simulink model "Smart_City_QCar2_VIRTUAL_car4"  (R2024b)
settings: Solver=ode1  StartTime=0.0  StopTime=inf  FixedStep=Controller_Sample_Time  RelTol=1e-3  EnableMultiTasking=on
values from neighbouring files (symbols this model uses):
  Audio_Sample_Time = 0.3    [Setup_QCar1and2_params.m]
  cameraStepSize = 3e-2    (= 0.03)    [Setup_QCar1and2_params.m]
  CSI_Sample_Time = 1/60    (= 0.0166666666667)    [Setup_QCar1and2_params.m]
  ImageDisplay_Sample_Time = CSI_Sample_Time*6    (= 0.1)    [Setup_QCar1and2_params.m]
  Initialization_Time = 5    [Setup_QCar1and2_params.m]
  LiDAR_Sample_Time = CSI_Sample_Time*3    (= 0.05)    [Setup_QCar1and2_params.m]
  map_mask = [1 1 1 0 0 1 0]    [Setup_QCar1and2_params.m]
  NN_Sample_Time = RealSense_Sample_Time*1    (= 0.0333333333333)    [Setup_QCar1and2_params.m]
  path_x = [0.826 0.836 0.846 0.856 0.866 0.876 0.886 0.896 0.906 0.916 0.926 0.936 ... (740 elements, 740x1)]    [SDCS_Paths_7.mat]
  path_x2 = [-0.614 -0.604 -0.594 -0.584 -0.574 -0.564 -0.554 -0.544 -0.534 -0.524 -0.514 -0.504 ... (1090 elements, 1090x1)]    [SDCS_Paths_7.mat]
  path_x3 = [-0.614 -0.603821428571 -0.593642857143 -0.583464285714 -0.573285714286 -0.563107142857 -0.552928571429 -0.54275 -0.532571428571 -0.522392857143 -0.512214285714 -0.502035714286 ... (714 elements, 714x1)]    [SDCS_Paths_7.mat]
  path_x4 = [-0.614 -0.604 -0.594 -0.584 -0.574 -0.564 -0.554 -0.544 -0.534 -0.524 -0.514 -0.504 ... (1761 elements, 1761x1)]    [SDCS_Paths_7.mat]
  path_x5 = [1.436 1.42588571429 1.41577142857 1.40565714286 1.39554285714 1.38542857143 1.37531428571 1.3652 1.35508571429 1.34497142857 1.33485714286 1.32474285714 ... (574 elements, 574x1)]    [SDCS_Paths_7.mat]
  path_x6 = [1.436 1.42588571429 1.41577142857 1.40565714286 1.39554285714 1.38542857143 1.37531428571 1.3652 1.35508571429 1.34497142857 1.33485714286 1.32474285714 ... (1288 elements, 1288x1)]    [SDCS_Paths_7.mat]
  path_x7 = [-1.5778487585 -1.56959877056 -1.56127865467 -1.55288878259 -1.54442952915 -1.53590127231 -1.52730439309 -1.51863927561 -1.50990630701 -1.50110587746 -1.49223838016 -1.4833042113 ... (2260 elements, 2260x1)]    [SDCS_Paths_7.mat]
  path_y = [-1.0887 -1.0887 -1.0887 -1.0887 -1.0887 -1.0887 -1.0887 -1.0887 -1.0887 -1.0887 -1.0887 -1.0887 ... (740 elements, 740x1)]    [SDCS_Paths_7.mat]
  path_y2 = [-1.0887 -1.0887 -1.0887 -1.0887 -1.0887 -1.0887 -1.0887 -1.0887 -1.0887 -1.0887 -1.0887 -1.0887 ... (1090 elements, 1090x1)]    [SDCS_Paths_7.mat]
  path_y3 = [-1.0887 -1.0887 -1.0887 -1.0887 -1.0887 -1.0887 -1.0887 -1.0887 -1.0887 -1.0887 -1.0887 -1.0887 ... (714 elements, 714x1)]    [SDCS_Paths_7.mat]
  path_y4 = [-1.0887 -1.0887 -1.0887 -1.0887 -1.0887 -1.0887 -1.0887 -1.0887 -1.0887 -1.0887 -1.0887 -1.0887 ... (1761 elements, 1761x1)]    [SDCS_Paths_7.mat]
  path_y5 = [-0.8157 -0.8157 -0.8157 -0.8157 -0.8157 -0.8157 -0.8157 -0.8157 -0.8157 -0.8157 -0.8157 -0.8157 ... (574 elements, 574x1)]    [SDCS_Paths_7.mat]
  path_y6 = [-0.8157 -0.8157 -0.8157 -0.8157 -0.8157 -0.8157 -0.8157 -0.8157 -0.8157 -0.8157 -0.8157 -0.8157 ... (1288 elements, 1288x1)]    [SDCS_Paths_7.mat]
  path_y7 = [-0.614490295955 -0.61974988896 -0.624981792226 -0.630185771997 -0.635361595765 -0.640509032279 -0.645627851559 -0.6507178249 -0.655778724888 -0.660810325409 -0.665812401655 -0.670784730139 ... (2260 elements, 2260x1)]    [SDCS_Paths_7.mat]
  RealSense_Sample_Time = CSI_Sample_Time*2    (= 0.0333333333333)    [Setup_QCar1and2_params.m]
undefined symbols (not defined in the file or in its folder): DiscIntNeverNeededParam, gcbh, Joystick_Sample_Time, JPEG, qc_get_step_size, video_display_show
libraries: quarc_library x61, simulink_extras x9, simulink x5
(part 1 of 4)
settings Model: SimulationMode=external  ExtModeTrigDuration=10000  Creator=PKaram  LastModifiedBy=user
settings SolverCC: AlgebraicLoopSolver=TrustRegion  PositivePriorityOrder=on  AutoInsertRateTranBlk=on
settings DataIOCC: ReturnWorkspaceOutputs=off
settings DebuggingCC: ParameterPrecisionLossMsg=none  UnconnectedInputMsg=warning  UnconnectedOutputMsg=warning  UnconnectedLineMsg=warning  ArithmeticOperatorsInVariantConditions=warning
settings ModelReferenceCC: EnableRefExpFcnMdlSchedulingChecks=on
settings SFSimCC: SimUseLocalCustomCode=off  CustomCodeUndefinedFunction=UseInterfaceOnly
settings RTWCC: Description=QUARC Win64 Target Using Toolchain  SystemTargetFile=quarc_win64.tlc  TemplateMakefile=quarc_linux_nvidia_tmf  RTWUseLocalCustomCode=off  Toolchain=QUARC win64 | nmake (64-bit Windows)  BuildConfiguration=Faster Runs  GPUComputeCapability=3.5  DLArmComputeVersion=19.05
settings CodeAppCC: StateflowObjectComments=on
settings STFCustomTargetCC: TargetLangStandard=C99 (ISO)  ConcurrentExecutionCompliant=on  GRTInterface=on  UseToolchainInfoCompliant=on  SystemTargetFile=quarc_win64.tlc
settings GRTTargetCC: ParMdlRefBuildCompliant=off  CompOptLevelCompliant=off  CombineOutputUpdateFcns=off  MatFileLogging=off  CPPClassGenCompliant=off  GRTInterface=on  ExtMode=on  ExtModeMexFile=quarc_comm  ExtModeMexArgs='-w -d %d -uri %u -car_number 4','shmem://%m:1'
settings ConfigComp: CovMetricSettings=dswe

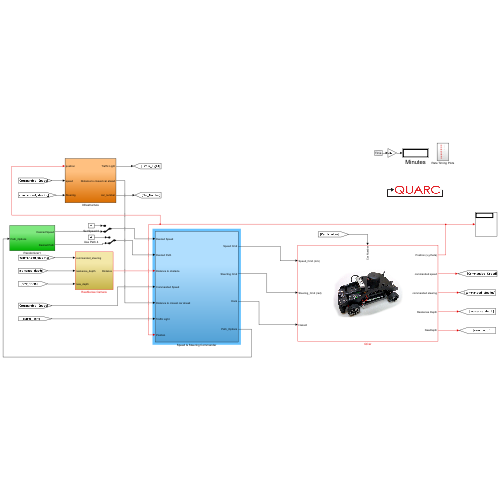
[thumbnail: Simulink's stored preview of the top-level diagram]
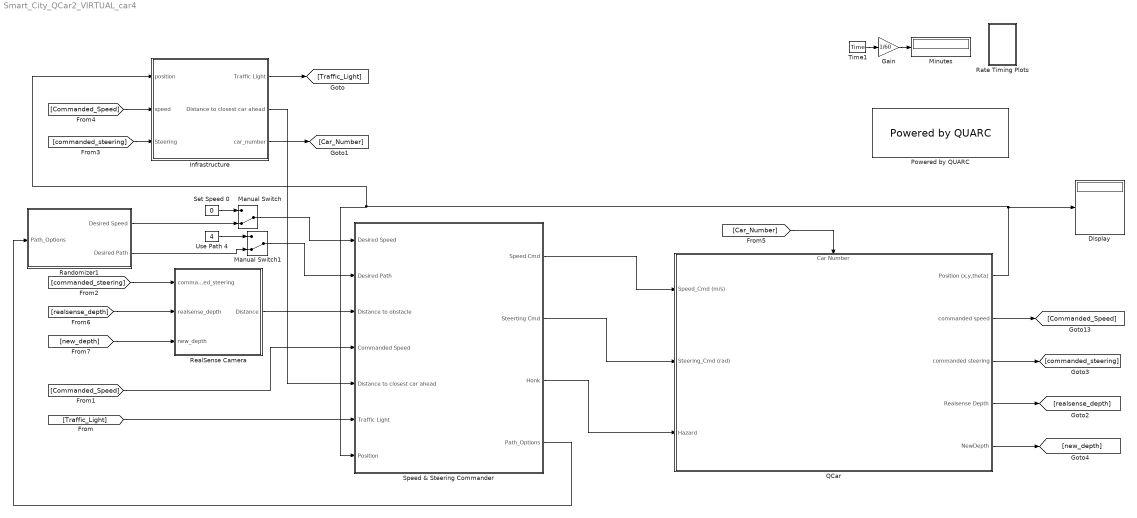
== system Smart_City_QCar2_VIRTUAL_car4 ==
  Display : Display
  Gain : Gain  Gain=1/60
  Infrastructure : Subsystem
  Manual Switch : ManualSwitch  CurrentSetting=0
  Manual Switch1 : ManualSwitch  CurrentSetting=0
  Minutes : Display
  Powered by QUARC : quarc_library/Logos/Powered by QUARC
  QCar : Subsystem
      settings: PortSchema="{\"entries\":[{\"content\":{\"sides\":[{\"content\":{\"connectorIds\":[\"In1\",\"In2\",\"In3\"]},\"type\":\"ConnectorPlacement.EquallySpacedRectSide\",\"uuid\":\"02a1560c-0405-4b97-a286-7d926425b90e\"},{\"content\":{\"connectorIds\":[\"Out1\",\"Out2\",\"Out3\",\"Out4\",\"Out5\"],\"side\":\"RIGHT\"},\"type\":\"ConnectorPlacement.EquallySpacedRectSide\",\"uuid\":\"39c5c8b2-4245-4ec7-b5b3-4c98e6a2673a\"},{\"content\":{\"connectorIds\":[\"In4\"],\"side\":\"TOP\"},\"type\":\"ConnectorPlacement.EquallySpacedRectSide\",\"uuid\":\"1752f2f8-f0ed-4d28-b225-c74112047425\"}]},\"type\":\"ConnectorPlacement.EquallySpacedConnector\",\"uuid\":\"d58cf7e2-2005-4c93-8747-d53ee0601380\"}],\"packageUris\":[\"http://schema.mathworks.com/mf0/Connector/R2020b\"],\"version\":\"1.0\"}"
      mask Display: image('QCar.png', [0,0,0,0,50,50]);
  Randomizer1 : Subsystem
  Rate Timing Plots : Subsystem
  RealSense Camera : Subsystem
  Set Speed 0 : Constant  Value=0
  Speed & Steering Commander : Subsystem
  Time1 : quarc_library/Sources/Time/Time  time_source=Wall clock  sample_time=qc_get_step_size
  Use Path 4 : Constant  Value=4
  wires:
  [commanded_steering] -> RealSense Camera/1(commanded_steering)
  [commanded_steering] -> Infrastructure/3(Steering)
  Use Path 4/1 -> Manual Switch1/1
  QCar/1(Position (x,y,theta)) -> Speed & Steering Commander/7(Position), Infrastructure/1(position), Display/1
  [Traffic_Light] -> Speed & Steering Commander/6(Traffic Light)
  QCar/3(commanded steering) -> [commanded_steering]
  Randomizer1/1(Desired Speed) -> Manual Switch/2
  [Commanded_Speed] -> Speed & Steering Commander/4(Commanded Speed)
  Time1/1 -> Gain/1
  Manual Switch/1 -> Speed & Steering Commander/1(Desired Speed)
  Manual Switch1/1 -> Speed & Steering Commander/2(Desired Path)
  Speed & Steering Commander/2(Steerting Cmd) -> QCar/2(Steering_Cmd (rad))
  Infrastructure/2(Distance to closest car ahead) -> Speed & Steering Commander/5(Distance to closest car ahead)
  Speed & Steering Commander/1(Speed Cmd) -> QCar/1(Speed_Cmd (m/s))
  Speed & Steering Commander/4(Path_Options) -> Randomizer1/1(Path_Options)
  Speed & Steering Commander/3(Honk) -> QCar/3(Hazard)
  Infrastructure/3(car_number) -> [Car_Number]
  QCar/2(commanded speed) -> [Commanded_Speed]
  Set Speed 0/1 -> Manual Switch/1
  [Commanded_Speed] -> Infrastructure/2("speed ")
  Randomizer1/2(Desired Path) -> Manual Switch1/2
  Gain/1 -> Minutes/1
  RealSense Camera/1(Distance) -> Speed & Steering Commander/3(Distance to obstacle)
  [Car_Number] -> QCar/4(Car Number)
  QCar/4(Realsense Depth) -> [realsense_depth]
  [realsense_depth] -> RealSense Camera/2(realsense_depth)
  QCar/5(NewDepth) -> [new_depth]
  [new_depth] -> RealSense Camera/3(new_depth)
  Infrastructure/1(Traffic Light) -> [Traffic_Light]

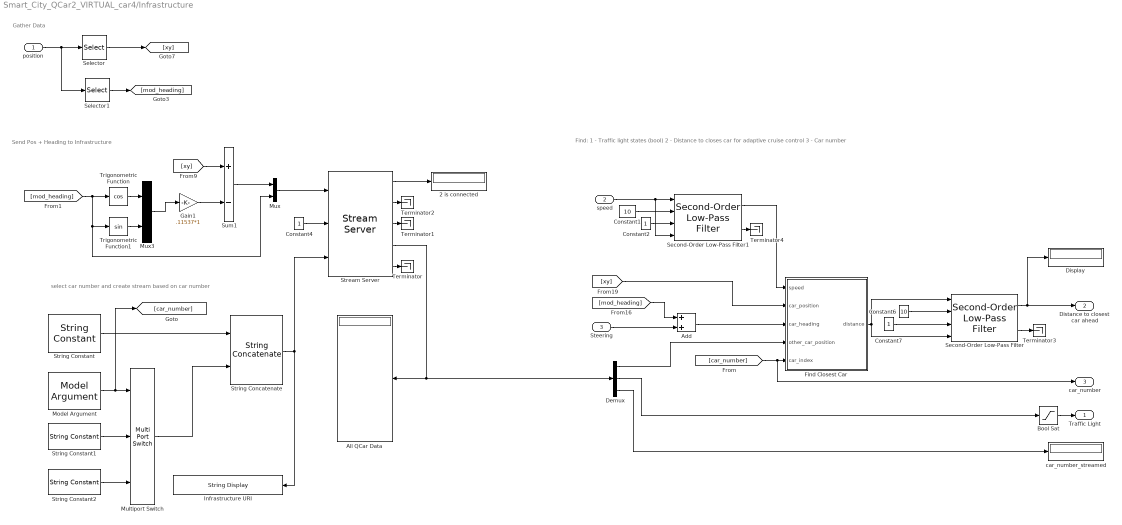
== system Smart_City_QCar2_VIRTUAL_car4/Infrastructure ==
  note: select car number and create stream based on car number
  note: Find:
      | 1 - Traffic light states (bool)
      | 2 - Distance to closes car for adaptive cruise control
      | 3 - Car number
  note: Send Pos + Heading to Infrastructure
  note: Gather Data
  position : Inport
  "speed " : Inport  Port=2
  Steering : Inport  Port=3
  2 is connected : Display
      settings: Decimation=100
  Add : Sum
  All QCar Data : Display
  Bool Sat : Saturate  UpperLimit=1  LowerLimit=0
  Constant1 : Constant  Value=10
  Constant2 : Constant
  Constant4 : Constant
  Constant6 : Constant  Value=10
  Constant7 : Constant
  Demux : Demux  Outputs=[10 1 1]
  Display : Display
  Find Closest Car : Subsystem
  Gain1 : Gain  Gain=.11537*1
  Infrastructure URI : quarc_library/Strings/String Display  alignment=center  display_mode=Single line  sample_time=-1  use_new=off
      settings: SourceProductName=QUARC Targets
  Model Argument : quarc_library/Sources/Signals/Model Argument  argument_name=car_number  has_value=on  data_type_mode=Specify via dialog  data_type=uint8  max_length=80  default_value=0  default_string=4  variable_size=on
      settings: AttributesFormatString=(-%<argument_name>)  SourceProductName=QUARC Targets
  Multiport Switch : MultiPortSwitch  DataPortOrder=Specify indices  DataPortIndices={4,5}  SaturateOnIntegerOverflow=off  InputSameDT=off
  Mux : Mux  Inputs=2
  Mux3 : Mux  Inputs=2
  Second-Order Low-Pass Filter : quarc_library/Continuous/Second-Order Low-Pass Filter  params_source=External (input ports)  input_width=1  input_zeta=1  input_init=0
  Second-Order Low-Pass Filter1 : quarc_library/Continuous/Second-Order Low-Pass Filter  params_source=External (input ports)  input_width=1  input_zeta=1  input_init=0
  Selector : Selector  InputPortWidth=3  IndexOptions=Index vector (dialog)  Indices=1:2  OutputSizes=1
  Selector1 : Selector  InputPortWidth=3  IndexOptions=Index vector (dialog)  Indices=3  OutputSizes=1
  Stream Server : quarc_library/Communications/Basic/Stream Server  uri_source=External input port  uri=tcpip://localhost:4444?nagle='off'  send_buffer_size=1460  receive_buffer_size=1460  byte_order=little endian (Intel - LSB first)  optimization=Minimum latency  send_options=Send most recent data  receive_options=Receive most recent data  default_value=10* ones (1,12)  sample_time=qc_get_step_size  active=off  implementation=Use blocking I/O in a separate thread  send_fifo_size=1  receive_fifo_size=1  send_priority=0  receive_priority=0  send_dimensions=off  receive_dimensions=off  max_dimensions=-1  data_type=Inherited via back propagation  type_expr=BusObject
  String Concatenate : quarc_library/Strings/String Concatenate  num_inputs=2  max_length=0  output_size=Inherit from input
      settings: SourceProductName=QUARC Targets
  String Constant : quarc_library/Strings/String Constant  string_value=tcpip://localhost:  evaluate_string=off  string_type=text  max_length=80  sample_time=inf  variable_size=off
      settings: AttributesFormatString="\"tcpip://localhost:\""  SourceProductName=QUARC Targets
  String Constant1 : quarc_library/Strings/String Constant  string_value=4444  evaluate_string=off  string_type=text  max_length=80  sample_time=inf  variable_size=off
      settings: AttributesFormatString="\"4444\""  SourceProductName=QUARC Targets
  String Constant2 : quarc_library/Strings/String Constant  string_value=5555  evaluate_string=off  string_type=text  max_length=80  sample_time=inf  variable_size=off
      settings: AttributesFormatString="\"5555\""  SourceProductName=QUARC Targets
  Sum1 : Sum  Inputs=+-
  Terminator{,1..4} (5 alike) : Terminator
  Trigonometric Function : Trigonometry  Operator=cos
  Trigonometric Function1 : Trigonometry
  car_number_streamed : Display
  Traffic Light : Outport
  Distance to closest car ahead : Outport  Port=2
  car_number : Outport  Port=3
  wires:
  Constant7/1 -> Second-Order Low-Pass Filter/3
  Constant4/1 -> Stream Server/2
  Stream Server/1 -> 2 is connected/1
  Constant6/1 -> Second-Order Low-Pass Filter/2
  position/1 -> Selector1/1, Selector/1
  Selector/1 -> [xy]
  Selector1/1 -> [mod_heading]
  Second-Order Low-Pass Filter/1 -> Display/1, Distance to closest car ahead/1
  Constant1/1 -> Second-Order Low-Pass Filter1/2
  "speed "/1 -> Second-Order Low-Pass Filter1/4, Second-Order Low-Pass Filter1/1
  Stream Server/4 -> All QCar Data/1, Demux/1
  [xy] -> Find Closest Car/2(car_position)
  Constant2/1 -> Second-Order Low-Pass Filter1/3
  Second-Order Low-Pass Filter1/1 -> Find Closest Car/1("speed ")
  Find Closest Car/1(distance) -> Second-Order Low-Pass Filter/1, Second-Order Low-Pass Filter/4
  Add/1 -> Find Closest Car/3(car_heading)
  [mod_heading] -> Add/1
  Steering/1 -> Add/2
  Demux/1 -> Find Closest Car/4(other_car_position)
  Demux/2 -> Bool Sat/1
  Bool Sat/1 -> Traffic Light/1
  Mux/1 -> Stream Server/1
  Sum1/1 -> Mux/1
  Demux/3 -> car_number_streamed/1
  [mod_heading] -> Mux/2, Trigonometric Function1/1, Trigonometric Function/1
  Mux3/1 -> Gain1/1
  Trigonometric Function1/1 -> Mux3/2
  [xy] -> Sum1/1
  Gain1/1 -> Sum1/2
  Trigonometric Function/1 -> Mux3/1
  Stream Server/5 -> Terminator/1
  Stream Server/3 -> Terminator1/1
  Stream Server/2 -> Terminator2/1
  Second-Order Low-Pass Filter/2 -> Terminator3/1
  Second-Order Low-Pass Filter1/2 -> Terminator4/1
  String Constant/1 -> String Concatenate/1
  Model Argument/1 -> [car_number], Multiport Switch/1
  String Constant1/1 -> Multiport Switch/2
  String Constant2/1 -> Multiport Switch/3
  Multiport Switch/1 -> String Concatenate/2
  String Concatenate/1 -> Stream Server/3, Infrastructure URI/1
  [car_number] -> car_number/1, Find Closest Car/5(car_index)

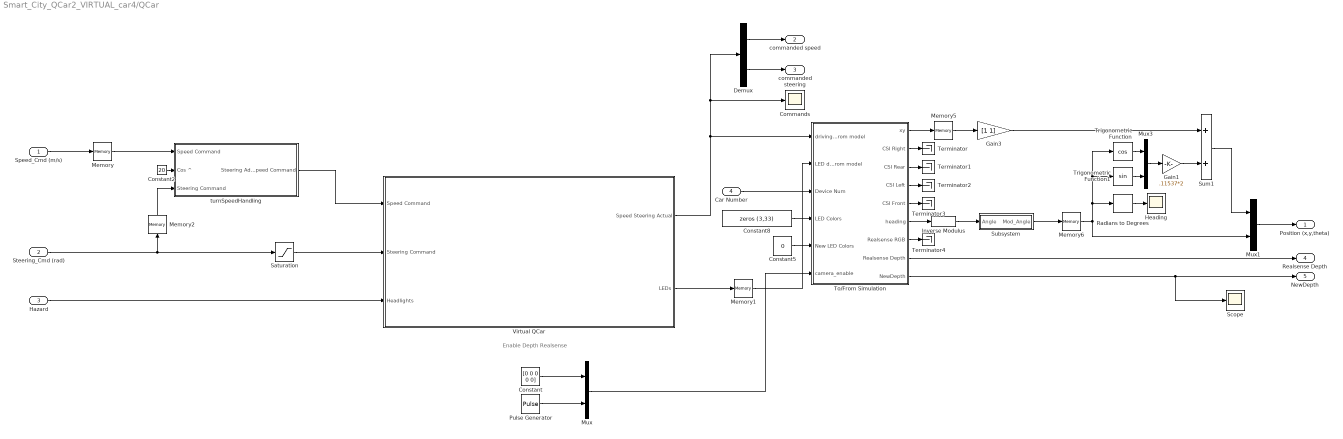
== system Smart_City_QCar2_VIRTUAL_car4/QCar ==
  note: Enable Depth Realsense
  Speed_Cmd (m/s) : Inport
  Steering_Cmd (rad) : Inport  Port=2
  Hazard : Inport  Port=3
  Car Number : Inport  Port=4
  Commands : Scope
  Constant : Constant  Value=[0 0 0 0 0]  SampleTime=RealSense_Sample_Time
  Constant2 : Constant  Value=20
  Constant5 : Constant  Value=0
  Constant8 : Constant  Value=zeros (3,33)
  Demux : Demux  Outputs=2
  Gain1 : Gain  Gain=.11537*2
  Gain3 : Gain  Gain=[1 1]
  Heading : Scope
  Inverse Modulus : quarc_library/Discontinuities/Inverse Modulus  modulus=2*pi  output_derivative=off  output_revolutions=off  max_x=Inf  min_x=-Inf
  Memory : Memory
  Memory1 : Memory  InitialCondition=zeros (1,16)  InheritSampleTime=on  LinearizeMemory=on  LinearizeAsDelay=on
  Memory2 : Memory  InheritSampleTime=on  LinearizeMemory=on  LinearizeAsDelay=on
  Memory5 : Memory  InitialCondition=[0 0]  InheritSampleTime=on  LinearizeMemory=on  LinearizeAsDelay=on
  Memory6 : Memory  InheritSampleTime=on  LinearizeMemory=on  LinearizeAsDelay=on
  Mux : Mux  Inputs=2
  Mux1 : Mux  Inputs=2
  Mux3 : Mux  Inputs=2
  Pulse Generator : DiscretePulseGenerator  SampleTime=RealSense_Sample_Time
  Radians to Degrees : simulink_extras/Transformations/Radians to Degrees
  Saturation : Saturate  UpperLimit=0.6  LowerLimit=-0.6
  Scope : Scope
  Subsystem : Subsystem
  Sum1 : Sum
  Terminator{,1..4} (5 alike) : Terminator
  To/From Simulation : Subsystem
  Trigonometric Function : Trigonometry  Operator=cos
  Trigonometric Function1 : Trigonometry
  Virtual QCar : Subsystem
  turnSpeedHandling : Subsystem
  Position (x,y,theta) : Outport
  commanded speed : Outport  Port=2
  commanded steering : Outport  Port=3
  Realsense Depth : Outport  Port=4
  NewDepth : Outport  Port=5
  wires:
  Saturation/1 -> Virtual QCar/2(Steering Command)
  Memory6/1 -> Mux1/2, Trigonometric Function/1, Trigonometric Function1/1, Radians to Degrees/1
  Subsystem/1(Mod_Angle) -> Memory6/1
  Memory5/1 -> Gain3/1
  turnSpeedHandling/1(Steering Adjusted Speed Command) -> Virtual QCar/1(Speed Command)
  Hazard/1 -> Virtual QCar/3(Headlights)
  Mux1/1 -> Position (x,y,theta)/1
  Sum1/1 -> Mux1/1
  Memory2/1 -> turnSpeedHandling/3(Steering Command)
  Constant2/1 -> turnSpeedHandling/2(Cos ^)
  Car Number/1 -> To/From Simulation/3(Device Num)
  Gain3/1 -> Sum1/1
  Gain1/1 -> Sum1/2
  Mux3/1 -> Gain1/1
  Trigonometric Function1/1 -> Mux3/2
  Trigonometric Function/1 -> Mux3/1
  Radians to Degrees/1 -> Heading/1
  Inverse Modulus/1 -> Subsystem/1(Angle)
  Virtual QCar/1(Speed Steering Actual) -> Demux/1, Commands/1, To/From Simulation/1(driving data from model)
  Virtual QCar/2(LEDs) -> Memory1/1
  Demux/1 -> commanded speed/1
  Constant8/1 -> To/From Simulation/4(LED Colors)
  Constant5/1 -> To/From Simulation/5(New LED Colors)
  To/From Simulation/6(heading) -> Inverse Modulus/1
  To/From Simulation/1(xy) -> Memory5/1
  Memory1/1 -> To/From Simulation/2(LED data from model)
  To/From Simulation/8(Realsense Depth) -> Realsense Depth/1
  Speed_Cmd (m/s)/1 -> Memory/1
  Memory/1 -> turnSpeedHandling/1(Speed Command)
  Steering_Cmd (rad)/1 -> Memory2/1, Saturation/1
  To/From Simulation/2(CSI Right) -> Terminator/1
  To/From Simulation/3(CSI Rear) -> Terminator1/1
  To/From Simulation/4(CSI Left) -> Terminator2/1
  To/From Simulation/5(CSI Front) -> Terminator3/1
  To/From Simulation/7(Realsense RGB) -> Terminator4/1
  Demux/2 -> commanded steering/1
  Constant/1 -> Mux/1
  Mux/1 -> To/From Simulation/6(camera_enable)
  To/From Simulation/9(NewDepth) -> Scope/1, NewDepth/1
  Pulse Generator/1 -> Mux/2

== system Smart_City_QCar2_VIRTUAL_car4/Randomizer1 ==
  note: Tunable Params
  Path_Options : Inport
  Base Speed : Constant  Value=.35
  Display : Display
  Display1 : Display
  MATLAB Function : MATLAB Function  TreatAsAtomicUnit=on
  Manual Map Mask : Gain  Gain=[1 1 1 1 1 1 0]
  Memory1 : Memory  InitialCondition=2  InheritSampleTime=on  LinearizeMemory=on  LinearizeAsDelay=on
  Memory2 : Memory  InitialCondition=1  InheritSampleTime=on  LinearizeMemory=on  LinearizeAsDelay=on
  Path 4 : Constant  Value=4
  Start on path 4 : Switch  Criteria=u2 > Threshold  Threshold=8  SaturateOnIntegerOverflow=off  InputSameDT=off
  Subsystem1 : Subsystem
  Terminator : Terminator
  Time : quarc_library/Sources/Time/Time  time_source=Wall clock  sample_time=qc_get_step_size
  Time b/w Path Changes : Constant  Value=3
  Desired Speed : Outport
  Desired Path : Outport  Port=2
  wires:
  Memory1/1 -> MATLAB Function/1(Previous_Path)
  Memory2/1 -> MATLAB Function/2(Previous_Speed)
  Time b/w Path Changes/1 -> Subsystem1/1(Random Period)
  Subsystem1/1(RisingEdgeTrigger) -> MATLAB Function/5(randomize)
  Base Speed/1 -> MATLAB Function/4(Speed_Cmd_Base)
  MATLAB Function/2(Desired_Speed) -> Desired Speed/1, Memory2/1, Display1/1
  MATLAB Function/1(Desired_Path) -> Start on path 4/1, Memory1/1
  Path_Options/1 -> Manual Map Mask/1
  MATLAB Function/3(Accel_Limit) -> Terminator/1
  Time/1 -> Start on path 4/2
  Start on path 4/1 -> Display/1, Desired Path/1
  Path 4/1 -> Start on path 4/3
  Manual Map Mask/1 -> MATLAB Function/3(Path_Options)

== system Smart_City_QCar2_VIRTUAL_car4/Rate Timing Plots ==
  Audio : Scope
  CSI : Scope
  Control : Scope
  Image Displays : Scope
  Joystick : Scope  Commented=on
  LCD : Scope
  LiDAR : Scope
  NN Rate : Scope
  RealSense : Scope
  monitorTiming : Subsystem
  monitorTiming1 : Subsystem
  monitorTiming2 : Subsystem
  monitorTiming3 : Subsystem
  monitorTiming4 : Subsystem  Commented=on
  monitorTiming5 : Subsystem
  monitorTiming6 : Subsystem
  monitorTiming7 : Subsystem
  monitorTiming8 : Subsystem
  wires:
  monitorTiming/1(Timing (s)) -> CSI/1
  monitorTiming1/1(Timing (s)) -> Control/1
  monitorTiming3/1(Timing (s)) -> Image Displays/1
  monitorTiming4/1(Timing (s)) -> Joystick/1
  monitorTiming2/1(Timing (s)) -> RealSense/1
  monitorTiming5/1(Timing (s)) -> LiDAR/1
  monitorTiming6/1(Timing (s)) -> NN Rate/1
  monitorTiming7/1(Timing (s)) -> LCD/1
  monitorTiming8/1(Timing (s)) -> Audio/1

== system Smart_City_QCar2_VIRTUAL_car4/RealSense Camera ==
  note: Capture Realsense and do Object Detection
  commanded_steering : Inport
  realsense_depth : Inport  Port=2
  new_depth : Inport  Port=3
  Constant8 : Constant  Value=50
  Constant9 : Constant
  Distance to Object Detected : Display
  Gain : Gain  Gain=3.9/255
  Image Transform : quarc_library/Image Processing/Generic/Image Transform  algorithm=Colorize  color_theme=KRYGCBMW  min_pixel=0  max_pixel=5  contour_depth=1  focal_length=308  principal_point=[262 334]  radial_coeffs=[-0.3129 0.0907]  tangential_coeffs=[]  extrapolated_pixel=0  interpolation=nearest  row_coords=0  column_coords=0  output_height=480  output_width=640  angle=0  origin=[240 320]  output_origin=[240 320]  output_data_type=uint8
      settings: AttributesFormatString=(%<algorithm>)  SourceProductName=QUARC Targets
  Newer Depth : Subsystem  LoadFcn=set_param(gcbh, 'UserData', gcb);  StartFcn=video_display_show([gcb, '/Video Display'], 'add', gcb);  mask(Video Compressed Display){algorithm=JPEG, quality=50, sample_time=-1, use_hardware=on}
      mask prompts: algorithm "Compression algorithm:"; quality "Compression quality (0-100):"; sample_time "Sample time (seconds):"; use_hardware "Use hardware acceleration for video display"
      mask help: Displays a video stream on the host, using compression to minimize bandwidth.
      mask init:
      | qc_set_display('Video\nCompressed\nDisplay');
      settings: UndoDeleteFcn=set_param(gcbh, 'UserData', gcb);  OpenFcn=video_display_show([gcb, '/Video Display'], 'show', gcb);  PreDeleteFcn=video_display_show([gcb, '/Video Display'], 'delete');
      settings: CopyFcn=|
      | set_param(gcbh, 'UserData', gcb);
      | set_param(gcbh, 'LinkStatus', 'none');
      settings: NameChangeFcn=|
      | video_display_show([get_param(gcbh, 'UserData'), '/Video Display'], 'rename', [gcb, '/Video Display']);
      | video_display_show([gcb, '/Video Display'], 'add', gcb);
      | set_param(gcbh, 'UserData', gcb);
      mask Help: web(qc_get_block_help_path(gcb));
      mask TypeOptions algorithm: Image Compress/algorithm
      mask TypeOptions quality: Image Compress/quality
      mask TypeOptions sample_time: Video Display/sample_time
      mask TypeOptions use_hardware: Video Display/use_hardware
      mask Display:
      | patch([0.98591 0.98591 0.62618 0.59072 0.56147   0.536   0.536  0.5441 0.56912 0.59207 0.60881 0.62276 0.63527 0.64364  0.6485  0.6485 0.64706 0.64499 0.63662 0.62411 0.61232 0.59837 0.58307 0.56147   0.536   0.536  0.5441  0.5747 0.60953 0.63662 0.67001  0.7034 0.72851 0.75425 0.77927 0.80294 0.82454 0.84119 0.85865 0.87395 0.88574 0.89339  0.8969 0.89969 0.89969 0.89267  0.8816 0.87044 0.85649  0.8384 0.81824 0.80294 0.78764 0.77513 0.76676 0.75776 0.76397 0.77513 0.79178 0.80987 0.82796 0.84326 0.86207 0.98528],[0.18689 0.05522 0.05522 0.05171 0.05171    0.05 0.18338 0.18338 0.19148 0.20435 0.22298 0.24863 0.28589 0.33125 0.38138 0.55139 0.59801 0.63761 0.68189 0.72149 0.74939 0.76694 0.77855 0.79367 0.79952 0.92768 0.92768 0.92768 0.92417 0.92066 0.91364  0.9032 0.89384 0.88106 0.86594 0.85073 0.82634 0.80537 0.77855 0.74363 0.70403 0.65858 0.61079 0.59099 0.41513 0.37202 0.31847 0.29048 0.25556 0.23342  0.2102 0.19382 0.18221 0.17285 0.16943 0.16124  0.1589 0.16241 0.16709 0.17168  0.1787 0.18221 0.18689 0.18689],[0.9,0.90,0.91])
      | patch([0.536 0.52601 0.46823 0.44528 0.41603 0.39101 0.35555 0.33116 0.31451 0.29291  0.2804 0.26717 0.25322 0.23999 0.22406 0.20732 0.19337 0.17528 0.15935 0.14396 0.13217 0.11759 0.10922 0.10085 0.09671 0.09392 0.09041 0.08906 0.08906 0.09464  0.0995 0.10778 0.11894 0.13145 0.14675 0.16349 0.17672 0.19409 0.20732 0.22406 0.23999 0.26159 0.27833 0.29849 0.31793 0.33602 0.35411 0.37085 0.39245 0.41603   0.536   0.536 0.53159 0.46409   0.446 0.42026 0.39587 0.37571 0.36113 0.34925 0.34088 0.33809 0.33809 0.34088 0.34583 0.35627 0.36392 0.38129 0.39587 0.41117 0.42719 0.44672  0.4676 0.48353 0.48353 0.52394   0.536],[0.05 0.04829 0.04712 0.04712 0.04829 0.05063 0.05405 0.05873 0.06107 0.06692 0.07043 0.07619 0.08087 0.08672 0.09482 0.10652 0.11696 0.13325  0.1508 0.17168 0.19499 0.22415 0.25439 0.28472 0.31379 0.35456 0.38489 0.41513 0.58055 0.63878 0.68774 0.72149 0.75641 0.78089 0.80537 0.82859 0.84029 0.85658 0.86594 0.87404  0.8834 0.89267 0.90086 0.90788 0.91247 0.91832 0.92066   0.923 0.92651 0.92768 0.92768 0.79952 0.79952 0.79952 0.79718 0.78899 0.77153 0.75056 0.72149 0.68072 0.62249  0.5549 0.41396 0.37085 0.33242 0.28121 0.25205 0.22181 0.20552 0.19499 0.18572 0.18221 0.17753 0.17636 0.17753  0.1787  0.1787],[0.9,0.90,0.91])
      | disp('Video\nCompressed\nDisplay');
  Rate Transition : RateTransition
  Rate Transition2 : RateTransition
  Rate Transition4 : RateTransition
  Second-Order Low-Pass Filter2 : quarc_library/Continuous/Second-Order Low-Pass Filter  params_source=External (input ports)  input_width=1  input_zeta=1  input_init=0
  Terminator : Terminator
  Transfer Fcn : TransferFcn  Numerator=[10]  Denominator=[1 10]
  convert to double : DataTypeConversion  SaturateOnIntegerOverflow=off  RndMeth=Floor
  obstacleDetection Markham March 22 : Subsystem
  to 16Hz4 : RateTransition  OutPortSampleTime=ImageDisplay_Sample_Time
  Distance : Outport
  wires:
  Transfer Fcn/1 -> Rate Transition4/1
  commanded_steering/1 -> Transfer Fcn/1
  Constant9/1 -> Second-Order Low-Pass Filter2/3
  obstacleDetection Markham March 22/2(distance (m)) -> Rate Transition2/1, Distance to Object Detected/1
  Rate Transition2/1 -> Second-Order Low-Pass Filter2/4, Second-Order Low-Pass Filter2/1
  obstacleDetection Markham March 22/1(imageDepthForDisplay) -> to 16Hz4/1
  Second-Order Low-Pass Filter2/2 -> Terminator/1
  realsense_depth/1 -> convert to double/1
  Rate Transition4/1 -> obstacleDetection Markham March 22/2(steering (rad))
  Constant8/1 -> Second-Order Low-Pass Filter2/2
  Second-Order Low-Pass Filter2/1 -> Distance/1
  to 16Hz4/1 -> Image Transform/1
  new_depth/1 -> Rate Transition/1
  Rate Transition/1 -> obstacleDetection Markham March 22/Enable
  convert to double/1 -> Gain/1
  Gain/1 -> obstacleDetection Markham March 22/1(imageDepth)
  Image Transform/1 -> Newer Depth/1(In1)

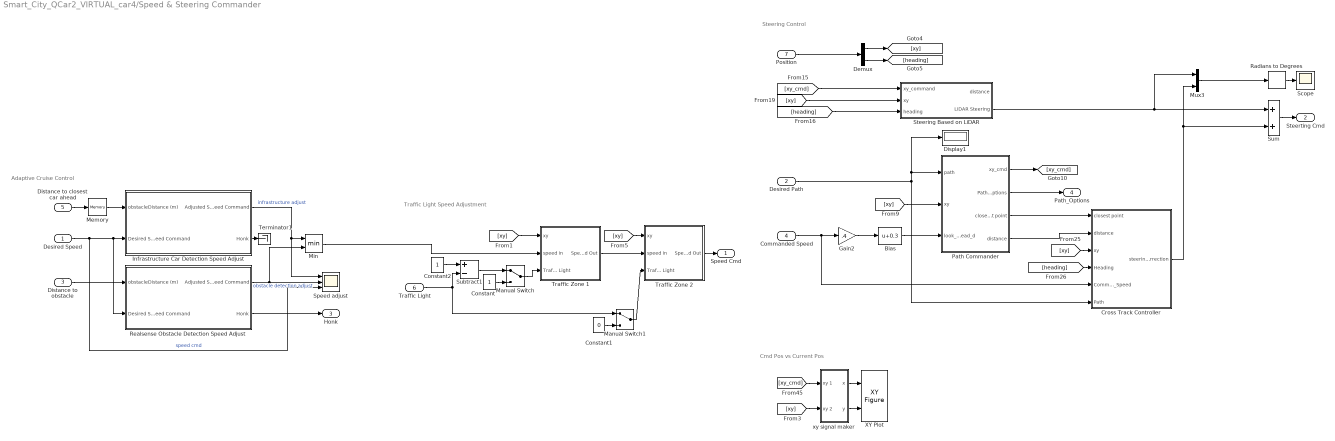
== system Smart_City_QCar2_VIRTUAL_car4/Speed & Steering Commander ==
  note: Steering Control
  note: Cmd Pos vs Current Pos
  note: Traffic Light Speed Adjustment
  note: Adaptive Cruise Control
  Desired Speed : Inport
  Desired Path : Inport  Port=2
  Distance to obstacle : Inport  Port=3
  Commanded Speed : Inport  Port=4
  Distance to closest car ahead : Inport  Port=5
  Traffic Light : Inport  Port=6
  Position : Inport  Port=7
  Bias : Bias  Bias=0.3  SaturateOnIntegerOverflow=off
  Constant : Constant
  Constant1 : Constant  Value=0
  Constant2 : Constant
  Cross Track Controller : Subsystem
  Demux : Demux  Outputs=2
  Display1 : Display
  Gain2 : Gain  Gain=.4
  Infrastructure Car Detection Speed Adjust : Subsystem
  Manual Switch : ManualSwitch
  Manual Switch1 : ManualSwitch
  Memory : Memory  InheritSampleTime=on  LinearizeMemory=on  LinearizeAsDelay=on
  Min : MinMax  Inputs=2
  Mux3 : Mux  Inputs=2
  Path Commander : Subsystem
  Radians to Degrees : simulink_extras/Transformations/Radians to Degrees
  Realsense Obstacle Detection Speed Adjust : Subsystem
  Scope : Scope
  Speed adjust : Scope  NumInputPorts=3
  Steering Based on LiDAR : Subsystem
  Subtract1 : Sum  Inputs=+-
  Sum : Sum
  Terminator1 : Terminator
  Traffic Zone 1 : Subsystem
  Traffic Zone 2 : Subsystem
  XY Plot : quarc_library/Sinks/Figures/XY Figure  figure_mode=Use figure window  figure_tag=figure1  axes_tag=axes1  plot_mode=Time-based  minimum_x=-2.5  maximum_x=2.5  minimum_y=-2  maximum_y=5  buffer_size=100  update_rate=1  initial_position="2   50  958  440"  initial_visibility=off  sample_time=-1
      settings: SourceProductName=QUARC Targets
  xy signal maker : Subsystem
  Speed Cmd : Outport
  Steerting Cmd : Outport  Port=2
  Honk : Outport  Port=3
  Path_Options : Outport  Port=4
  wires:
  [heading] -> Steering Based on LiDAR/3(heading)
  Bias/1 -> Path Commander/3(look_ahead_d)
  [xy] -> Cross Track Controller/3(xy)
  Gain2/1 -> Bias/1
  [heading] -> Cross Track Controller/4(Heading)
  Commanded Speed/1 -> Cross Track Controller/5(Commanded_Speed), Gain2/1
  [xy] -> Path Commander/2(xy)
  Mux3/1 -> Radians to Degrees/1
  [xy_cmd] -> Steering Based on LiDAR/1(xy_command)
  Desired Path/1 -> Display1/1, Path Commander/1(path), Cross Track Controller/6(Path)
  Steering Based on LiDAR/2(LiDAR Steering) -> Mux3/1, Sum/1
  [xy] -> Steering Based on LiDAR/2(xy)
  Path Commander/3(closest point) -> Cross Track Controller/1(closest point)
  Path Commander/1(xy_cmd) -> [xy_cmd]
  Cross Track Controller/1(steering correction) -> Mux3/2, Sum/2
  Radians to Degrees/1 -> Scope/1
  Path Commander/4(distance) -> Cross Track Controller/2(distance)
  Distance to obstacle/1 -> Realsense Obstacle Detection Speed Adjust/1(obstacleDistance (m))
  Desired Speed/1 -> Speed adjust/3, Infrastructure Car Detection Speed Adjust/2(Desired Speed Command), Realsense Obstacle Detection Speed Adjust/2(Desired Speed Command)  "speed cmd"
  Demux/2 -> [heading]
  Position/1 -> Demux/1
  Demux/1 -> [xy]
  Sum/1 -> Steerting Cmd/1
  Realsense Obstacle Detection Speed Adjust/2(Honk) -> Honk/1
  xy signal maker/2(y) -> XY Plot/2
  [xy_cmd] -> xy signal maker/1(xy 1)
  [xy] -> xy signal maker/2(xy 2)
  xy signal maker/1(x) -> XY Plot/1
  Traffic Zone 2/1(Speed Out) -> Speed Cmd/1
  Distance to closest car ahead/1 -> Memory/1
  Infrastructure Car Detection Speed Adjust/1(Adjusted Speed Command) -> Speed adjust/1, Min/1  "infrastructure adjust"
  Realsense Obstacle Detection Speed Adjust/1(Adjusted Speed Command) -> Min/2, Speed adjust/2  "obstacle detection adjust"
  Memory/1 -> Infrastructure Car Detection Speed Adjust/1(obstacleDistance (m))
  Path Commander/2(Path_Options) -> Path_Options/1
  Infrastructure Car Detection Speed Adjust/2(Honk) -> Terminator1/1
  Manual Switch/1 -> Traffic Zone 1/3(Traffic Light)
  Constant/1 -> Manual Switch/2
  Traffic Zone 1/1(Speed Out) -> Traffic Zone 2/2(speed in)
  Constant1/1 -> Manual Switch1/2
  [xy] -> Traffic Zone 1/1(xy)
  [xy] -> Traffic Zone 2/1(xy)
  Subtract1/1 -> Manual Switch/1
  Manual Switch1/1 -> Traffic Zone 2/3(Traffic Light)
  Constant2/1 -> Subtract1/1
  Traffic Light/1 -> Manual Switch1/1, Subtract1/2
  Min/1 -> Traffic Zone 1/2(speed in)

== system Smart_City_QCar2_VIRTUAL_car4/Infrastructure/Find Closest Car ==
  "speed " : Inport
  car_position : Inport  Port=2
  car_heading : Inport  Port=3
  other_car_position : Inport  Port=4
  car_index : Inport  Port=5
  Constant1 : Constant  Value=65
  Constant2 : Constant  Value=45
  Constant6 : Constant
  Constant7 : Constant
  Constant8 : Constant  Value=10
  Degrees to Radians : simulink_extras/Transformations/Degrees to Radians
  Demux : Demux  Outputs=2
  Demux1 : Demux  Outputs=2
  Display{,1..3} (4 alike) : Display
      settings: Decimation=100
  MATLAB Function : MATLAB Function  TreatAsAtomicUnit=on
  MATLAB Function1 : MATLAB Function  TreatAsAtomicUnit=on
  Radians to Degrees : simulink_extras/Transformations/Radians to Degrees
  Saturation Dynamic : simulink/Discontinuities/Saturation Dynamic  OutMin=[]  OutMax=[]  OutDataTypeStr=Inherit: Same as second input  OutDataType=fixdt(1, 16)  OutScaling=2^-10  DoSatur=off
  distance : Outport
  wires:
  Constant6/1 -> MATLAB Function/7(proximity_radius)
  Constant8/1 -> MATLAB Function/9(max_distance)
  car_index/1 -> MATLAB Function/5(car_index)
  Radians to Degrees/1 -> Display2/1
  car_heading/1 -> MATLAB Function/6(heading)
  MATLAB Function/2(distance_vector) -> Display1/1
  Degrees to Radians/1 -> MATLAB Function/8(proximity_scan_window)
  MATLAB Function/3(heading_vector) -> Radians to Degrees/1
  MATLAB Function/1(distance) -> Display/1, distance/1
  Demux/1 -> MATLAB Function/1(x_car)
  Demux/2 -> MATLAB Function/2(y_car)
  car_position/1 -> Demux/1
  other_car_position/1 -> Demux1/1
  Demux1/1 -> MATLAB Function/3(x_vector)
  Demux1/2 -> MATLAB Function/4(y_vector)
  "speed "/1 -> MATLAB Function1/1(speed)
  Constant7/1 -> MATLAB Function1/2(max_speed)
  Constant1/1 -> Saturation Dynamic/1, MATLAB Function1/4(max_window)
  Constant2/1 -> Saturation Dynamic/3, MATLAB Function1/3(min_window)
  MATLAB Function1/1(proximity_scan_window) -> Saturation Dynamic/2
  Saturation Dynamic/1 -> Display3/1, Degrees to Radians/1

== system Smart_City_QCar2_VIRTUAL_car4/QCar/Subsystem ==
  Angle : Inport
  Bias : Bias  Bias=pi  SaturateOnIntegerOverflow=off
  Bias1 : Bias  Bias=-pi  SaturateOnIntegerOverflow=off
  Constant1 : Constant  Value=2*pi
  Mod : Math  Operator=mod
  Mod_Angle : Outport
  wires:
  Angle/1 -> Bias/1
  Bias1/1 -> Mod_Angle/1
  Bias/1 -> Mod/1
  Constant1/1 -> Mod/2
  Mod/1 -> Bias1/1

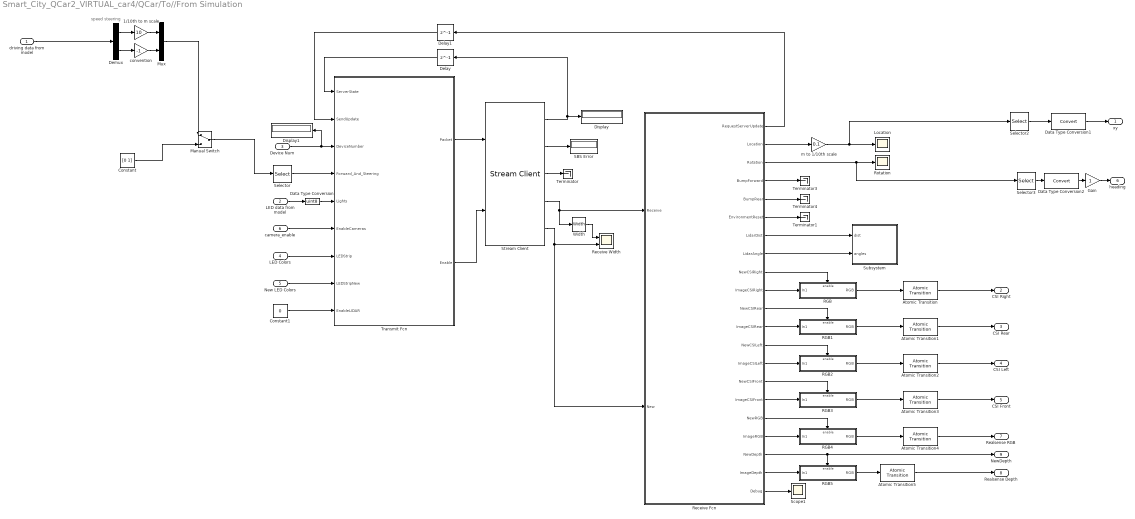
== system Smart_City_QCar2_VIRTUAL_car4/QCar/To//From Simulation ==
  note: speed
      | steering
  driving data from model : Inport
  LED data from model : Inport  Port=2
  Device Num : Inport  Port=3
  LED Colors : Inport  Port=4
  New LED Colors : Inport  Port=5
  camera_enable : Inport  Port=6
  1/10th to m scale : Gain  Gain=10
  Atomic Transition{,1..4} (5 alike) : quarc_library/Advanced/Asynchronous/Atomic Transition  sample_time=cameraStepSize  data_type=Inherit: Same as input
      settings: SourceProductName=QUARC Targets
  Atomic Transition5 : quarc_library/Advanced/Asynchronous/Atomic Transition  sample_time=RealSense_Sample_Time  data_type=Inherit: Same as input
      settings: SourceProductName=QUARC Targets
  Constant : Constant  Value=[0 1]
  Constant1 : Constant  Value=0
  Data Type Conversion : DataTypeConversion  OutDataTypeStr=uint8  SaturateOnIntegerOverflow=off  RndMeth=Floor
  Data Type Conversion1 : DataTypeConversion  SaturateOnIntegerOverflow=off  RndMeth=Floor
  Data Type Conversion2 : DataTypeConversion  SaturateOnIntegerOverflow=off  RndMeth=Floor
  Delay : Delay  DelayLength=1
  Delay1 : Delay  DelayLength=1
  Demux : Demux  Outputs=2
  Display : Display
  Display1 : Display
  Gain : Gain
  Location : Scope
  Manual Switch : ManualSwitch
  Mux : Mux  Inputs=2
  RGB : Subsystem
  RGB1 : Subsystem
  RGB2 : Subsystem
  RGB3 : Subsystem
  RGB4 : Subsystem
  RGB5 : Subsystem
  Receive Fcn : MATLAB Function  TreatAsAtomicUnit=on
  Receive Width : Scope  NumInputPorts=2
  Rotation : Scope
  SBS Error : Display
  Scope1 : Scope
  Selector : Selector  InputPortWidth=2  IndexOptions=Index vector (dialog)  Indices=[2 1]  OutputSizes=1
  Selector2 : Selector  InputPortWidth=3  IndexOptions=Index vector (dialog)  Indices=1:2  OutputSizes=1
  Selector3 : Selector  InputPortWidth=3  IndexOptions=Index vector (dialog)  Indices=3  OutputSizes=1
  Stream Client : quarc_library/Communications/Basic/Stream Client  uri_source=Specify via dialog (do not evaluate)  uri=tcpip://localhost:18000?nagle='off'  send_buffer_size=100000  receive_buffer_size=800000  byte_order=little endian (Intel - LSB first)  optimization=Minimum latency  send_options=Send all data  receive_options=Receive all data  default_value=[0]  sample_time=qc_get_step_size  active=on  implementation=Use blocking I/O in a separate thread  send_fifo_size=2  receive_fifo_size=2  send_priority=0  receive_priority=0  send_dimensions=on  receive_dimensions=on  max_dimensions=800000  data_type=uint8  type_expr=BusObject
      settings: AttributesFormatString="\"tcpip://localhost:18000?nagle='off'\""
  Subsystem : Subsystem
  Terminator{,1,3..4} (4 alike) : Terminator
  Transmit Fcn : MATLAB Function  TreatAsAtomicUnit=on
  Width : Width
  convention : Gain  Gain=-1
  m to 1/10th scale : Gain  Gain=0.1
  xy : Outport
  CSI Right : Outport  Port=2
  CSI Rear : Outport  Port=3
  CSI Left : Outport  Port=4
  CSI Front : Outport  Port=5
  heading : Outport  Port=6
  Realsense RGB : Outport  Port=7
  Realsense Depth : Outport  Port=8
  NewDepth : Outport  Port=9
  wires:
  New LED Colors/1 -> Transmit Fcn/8(LEDStripNew)
  LED Colors/1 -> Transmit Fcn/7(LEDStrip)
  LED data from model/1 -> Data Type Conversion/1
  Data Type Conversion/1 -> Transmit Fcn/5(Lights)
  Atomic Transition/1 -> CSI Right/1
  Receive Fcn/6(EnvironmentReset) -> Terminator1/1
  Stream Client/3 -> Terminator/1
  Stream Client/4 -> Receive Fcn/1(Receive), Width/1
  Transmit Fcn/1(Packet) -> Stream Client/1
  Receive Fcn/4(BumpForward) -> Terminator3/1
  Delay1/1 -> Transmit Fcn/2(SendUpdate)
  Receive Fcn/2(Location) -> m to 1/10th scale/1
  Atomic Transition1/1 -> CSI Rear/1
  RGB/1(RGB) -> Atomic Transition/1
  Receive Fcn/3(Rotation) -> Selector3/1, Rotation/1
  m to 1/10th scale/1 -> Location/1, Selector2/1
  Receive Fcn/11(NewCSIRear) -> RGB1/Enable
  Delay/1 -> Transmit Fcn/1(ServerState)
  Receive Fcn/14(ImageCSILeft) -> RGB2/1(In1)
  Receive Fcn/15(NewCSIFront) -> RGB3/Enable
  Stream Client/5 -> Receive Width/2, Receive Fcn/2(New)
  Stream Client/1 -> Delay/1, Display/1
  Atomic Transition3/1 -> CSI Front/1
  RGB2/1(RGB) -> Atomic Transition2/1
  Receive Fcn/18(ImageRGB) -> RGB4/1(In1)
  Receive Fcn/21(Debug) -> Scope1/1
  Receive Fcn/20(ImageDepth) -> RGB5/1(In1)
  Receive Fcn/7(LidarDist) -> Subsystem/1(dist)
  Atomic Transition2/1 -> CSI Left/1
  Stream Client/2 -> SBS Error/1
  Receive Fcn/1(RequestServerUpdate) -> Delay1/1
  RGB4/1(RGB) -> Atomic Transition4/1
  RGB1/1(RGB) -> Atomic Transition1/1
  Receive Fcn/5(BumpRear) -> Terminator4/1
  Receive Fcn/8(LidarAngle) -> Subsystem/2(angles)
  Receive Fcn/9(NewCSIRight) -> RGB/Enable
  Receive Fcn/16(ImageCSIFront) -> RGB3/1(In1)
  Receive Fcn/12(ImageCSIRear) -> RGB1/1(In1)
  Receive Fcn/13(NewCSILeft) -> RGB2/Enable
  RGB3/1(RGB) -> Atomic Transition3/1
  Receive Fcn/17(NewRGB) -> RGB4/Enable
  Width/1 -> Receive Width/1
  RGB5/1(RGB) -> Atomic Transition5/1
  Receive Fcn/10(ImageCSIRight) -> RGB/1(In1)
  Atomic Transition4/1 -> Realsense RGB/1
  Transmit Fcn/2(Enable) -> Stream Client/2
  Device Num/1 -> Display1/1, Transmit Fcn/3(DeviceNumber)
  convention/1 -> Mux/2
  Demux/1 -> 1/10th to m scale/1
  Demux/2 -> convention/1
  1/10th to m scale/1 -> Mux/1
  driving data from model/1 -> Demux/1
  Gain/1 -> heading/1
  Selector2/1 -> Data Type Conversion1/1
  Data Type Conversion2/1 -> Gain/1
  Selector3/1 -> Data Type Conversion2/1
  Data Type Conversion1/1 -> xy/1
  Manual Switch/1 -> Selector/1
  Mux/1 -> Manual Switch/1
  Constant/1 -> Manual Switch/2
  Selector/1 -> Transmit Fcn/4(Forward_And_Steering)
  Constant1/1 -> Transmit Fcn/9(EnableLIDAR)
  camera_enable/1 -> Transmit Fcn/6(EnableCameras)
  Receive Fcn/19(NewDepth) -> NewDepth/1, RGB5/Enable
  Atomic Transition5/1 -> Realsense Depth/1

== system Smart_City_QCar2_VIRTUAL_car4/QCar/Virtual QCar ==
  Speed Command : Inport
  Steering Command : Inport  Port=2
  Headlights : Inport  Port=3
  Constant1 : Constant  Value=.3
  Constant3 : Constant
  Constant4 : Constant  Value=2
  Constant5 : Constant  Value=-inf
  Electric Motor Model : Subsystem
  LED Logic : Subsystem
  Mux4 : Mux  Inputs=2
  Rate Limiter Dynamic : simulink/Discontinuities/Rate Limiter Dynamic
  Speed Controller Performance : Scope  NumInputPorts=2
  Transfer Fcn : TransferFcn  Denominator=[0.16 1]
  basicSpeedEstimation : Subsystem
  speedController : Subsystem
  Speed Steering Actual : Outport
  LEDs : Outport  Port=2
  wires:
  Constant1/1 -> Electric Motor Model/2(motor_limit)
  Transfer Fcn/1 -> Mux4/2, LED Logic/3(Steering)
  Constant5/1 -> Rate Limiter Dynamic/3
  Constant4/1 -> Rate Limiter Dynamic/1
  Rate Limiter Dynamic/1 -> Speed Controller Performance/1, speedController/2(desiredSpeed (m/s))
  LED Logic/1(LEDs) -> LEDs/1
  Mux4/1 -> Speed Steering Actual/1
  speedController/1(PWM Cmd) -> LED Logic/2(Throttle), Electric Motor Model/1(motor PWM Command (%))
  Electric Motor Model/1(Motor Speed (rad/s)) -> basicSpeedEstimation/1(motorSpeed (rad/s))
  basicSpeedEstimation/1(longitudinalCarSpeed (m/s)) -> LED Logic/1(Speed), Mux4/1, Speed Controller Performance/2, speedController/3(measuredSpeed (m/s))
  Constant3/1 -> speedController/1(arm (0,1))
  Steering Command/1 -> Transfer Fcn/1
  Speed Command/1 -> Rate Limiter Dynamic/2
  Headlights/1 -> LED Logic/4(Headlights)

== system Smart_City_QCar2_VIRTUAL_car4/QCar/turnSpeedHandling ==
  Speed Command : Inport
  Cos ^ : Inport  Port=2
  Steering Command : Inport  Port=3
  Cos : Trigonometry  Operator=cos
  Product : Product
  Saturation : Saturate  UpperLimit=1  LowerLimit=.3
  Scope : Scope  NumInputPorts=2
  Square : Math  Operator=pow  SignedPower=on
  Steering Adjusted Speed Command : Outport  VectorParamsAs1DForOutWhenUnconnected=off
  wires:
  Steering Command/1 -> Cos/1
  Product/1 -> Scope/2, Steering Adjusted Speed Command/1
  Square/1 -> Saturation/1
  Cos ^/1 -> Square/2
  Speed Command/1 -> Scope/1, Product/1  "Speed Command"
  Saturation/1 -> Product/2
  Cos/1 -> Square/1

== system Smart_City_QCar2_VIRTUAL_car4/Randomizer1/Subsystem1 ==
  Random Period : Inport
  Constant1 : Constant
  Less Than : RelationalOperator  Operator=<  OutDataTypeStr=boolean  RndMeth=Simplest  InputSameDT=off
  Mod : Math  Operator=mod
  Rate Transition : RateTransition  OutPortSampleTime=qc_get_step_size
  RisingEdge : Subsystem
  Time : quarc_library/Sources/Time/Time  time_source=Wall clock  sample_time=cameraStepSize*10
  RisingEdgeTrigger : Outport
  wires:
  Mod/1 -> Less Than/1
  Constant1/1 -> Less Than/2
  Rate Transition/1 -> Mod/1
  Less Than/1 -> RisingEdge/1(Input)
  Random Period/1 -> Mod/2
  Time/1 -> Rate Transition/1
  RisingEdge/1(RisingEdgeTrigger) -> RisingEdgeTrigger/1

== system Smart_City_QCar2_VIRTUAL_car4/Rate Timing Plots/monitorTiming ==
  note: Timing Performance
  note: moniorTiming Module:
      |
      | This subsystem outputs the sample time and computation time of the model.
      |
      | Outputs:
      | sampleTime (s) n/a : Sample time (unfiltered and filtered) in seconds.
      | computationTime (s) n/a : Computation time (unfiltered and filtered) in seconds.
      |
      | Usage:
      | Compare the Sample Time (s) output to a constant (qc_get_step_size) to monitor whether or not the desired sample time is being achieved. The Computation Time (s) values should be lower than the corresponding sample time value to ensure that the solver has enough time per time step.
  Computation Time : quarc_library/Sources/Time/Computation Time  sample_time=CSI_Sample_Time/2  use_model=on  use_cpu_time=off
  Constant : Constant  Value=CSI_Sample_Time/2  SampleTime=-1
  Mux : Mux  Inputs=3
  Sample Time : quarc_library/Sources/Time/Sample Time  Priority=-99  sample_time=CSI_Sample_Time/2
  Timing (s) : Outport  VectorParamsAs1DForOutWhenUnconnected=off
  wires:
  Computation Time/1 -> Mux/3
  Mux/1 -> Timing (s)/1
  Sample Time/1 -> Mux/1
  Constant/1 -> Mux/2

== system Smart_City_QCar2_VIRTUAL_car4/Rate Timing Plots/monitorTiming1 ==
  note: moniorTiming Module:
      |
      | This subsystem outputs the sample time and computation time of the model.
      |
      | Outputs:
      | sampleTime (s) n/a : Sample time (unfiltered and filtered) in seconds.
      | computationTime (s) n/a : Computation time (unfiltered and filtered) in seconds.
      |
      | Usage:
      | Compare the Sample Time (s) output to a constant (qc_get_step_size) to monitor whether or not the desired sample time is being achieved. The Computation Time (s) values should be lower than the corresponding sample time value to ensure that the solver has enough time per time step.
  note: Timing Performance
  Computation Time : quarc_library/Sources/Time/Computation Time  sample_time=qc_get_step_size  use_model=on  use_cpu_time=off
  Constant : Constant  Value=qc_get_step_size  SampleTime=-1
  Mux : Mux  Inputs=3
  Sample Time : quarc_library/Sources/Time/Sample Time  Priority=-99  sample_time=qc_get_step_size
  Timing (s) : Outport  VectorParamsAs1DForOutWhenUnconnected=off
  wires:
  Constant/1 -> Mux/2
  Sample Time/1 -> Mux/1
  Mux/1 -> Timing (s)/1
  Computation Time/1 -> Mux/3

== system Smart_City_QCar2_VIRTUAL_car4/Rate Timing Plots/monitorTiming2 ==
  note: moniorTiming Module:
      |
      | This subsystem outputs the sample time and computation time of the model.
      |
      | Outputs:
      | sampleTime (s) n/a : Sample time (unfiltered and filtered) in seconds.
      | computationTime (s) n/a : Computation time (unfiltered and filtered) in seconds.
      |
      | Usage:
      | Compare the Sample Time (s) output to a constant (qc_get_step_size) to monitor whether or not the desired sample time is being achieved. The Computation Time (s) values should be lower than the corresponding sample time value to ensure that the solver has enough time per time step.
  note: Timing Performance
  Computation Time : quarc_library/Sources/Time/Computation Time  sample_time=RealSense_Sample_Time  use_model=on  use_cpu_time=off
  Constant : Constant  Value=RealSense_Sample_Time  SampleTime=-1
  Mux : Mux  Inputs=3
  Sample Time : quarc_library/Sources/Time/Sample Time  Priority=-99  sample_time=RealSense_Sample_Time
  Timing (s) : Outport  VectorParamsAs1DForOutWhenUnconnected=off
  wires:
  Constant/1 -> Mux/2
  Sample Time/1 -> Mux/1
  Mux/1 -> Timing (s)/1
  Computation Time/1 -> Mux/3

== system Smart_City_QCar2_VIRTUAL_car4/Rate Timing Plots/monitorTiming3 ==
  note: Timing Performance
  note: moniorTiming Module:
      |
      | This subsystem outputs the sample time and computation time of the model.
      |
      | Outputs:
      | sampleTime (s) n/a : Sample time (unfiltered and filtered) in seconds.
      | computationTime (s) n/a : Computation time (unfiltered and filtered) in seconds.
      |
      | Usage:
      | Compare the Sample Time (s) output to a constant (qc_get_step_size) to monitor whether or not the desired sample time is being achieved. The Computation Time (s) values should be lower than the corresponding sample time value to ensure that the solver has enough time per time step.
  Computation Time : quarc_library/Sources/Time/Computation Time  sample_time=ImageDisplay_Sample_Time  use_model=on  use_cpu_time=off
  Constant : Constant  Value=ImageDisplay_Sample_Time  SampleTime=-1
  Mux : Mux  Inputs=3
  Sample Time : quarc_library/Sources/Time/Sample Time  Priority=-99  sample_time=ImageDisplay_Sample_Time
  Timing (s) : Outport  VectorParamsAs1DForOutWhenUnconnected=off
  wires:
  Computation Time/1 -> Mux/3
  Mux/1 -> Timing (s)/1
  Sample Time/1 -> Mux/1
  Constant/1 -> Mux/2

== system Smart_City_QCar2_VIRTUAL_car4/Rate Timing Plots/monitorTiming4 ==
  note: Timing Performance
  note: moniorTiming Module:
      |
      | This subsystem outputs the sample time and computation time of the model.
      |
      | Outputs:
      | sampleTime (s) n/a : Sample time (unfiltered and filtered) in seconds.
      | computationTime (s) n/a : Computation time (unfiltered and filtered) in seconds.
      |
      | Usage:
      | Compare the Sample Time (s) output to a constant (qc_get_step_size) to monitor whether or not the desired sample time is being achieved. The Computation Time (s) values should be lower than the corresponding sample time value to ensure that the solver has enough time per time step.
  Computation Time : quarc_library/Sources/Time/Computation Time  sample_time=Joystick_Sample_Time  use_model=on  use_cpu_time=off
  Constant : Constant  Value=Joystick_Sample_Time  SampleTime=-1
  Mux : Mux  Inputs=3
  Sample Time : quarc_library/Sources/Time/Sample Time  Priority=-99  sample_time=Joystick_Sample_Time
  Timing (s) : Outport  VectorParamsAs1DForOutWhenUnconnected=off
  wires:
  Computation Time/1 -> Mux/3
  Mux/1 -> Timing (s)/1
  Sample Time/1 -> Mux/1
  Constant/1 -> Mux/2

== system Smart_City_QCar2_VIRTUAL_car4/Rate Timing Plots/monitorTiming5 ==
  note: moniorTiming Module:
      |
      | This subsystem outputs the sample time and computation time of the model.
      |
      | Outputs:
      | sampleTime (s) n/a : Sample time (unfiltered and filtered) in seconds.
      | computationTime (s) n/a : Computation time (unfiltered and filtered) in seconds.
      |
      | Usage:
      | Compare the Sample Time (s) output to a constant (qc_get_step_size) to monitor whether or not the desired sample time is being achieved. The Computation Time (s) values should be lower than the corresponding sample time value to ensure that the solver has enough time per time step.
  note: Timing Performance
  Computation Time : quarc_library/Sources/Time/Computation Time  sample_time=LiDAR_Sample_Time  use_model=on  use_cpu_time=off
  Constant : Constant  Value=LiDAR_Sample_Time  SampleTime=-1
  Mux : Mux  Inputs=3
  Sample Time : quarc_library/Sources/Time/Sample Time  Priority=-99  sample_time=LiDAR_Sample_Time
  Timing (s) : Outport  VectorParamsAs1DForOutWhenUnconnected=off
  wires:
  Constant/1 -> Mux/2
  Sample Time/1 -> Mux/1
  Mux/1 -> Timing (s)/1
  Computation Time/1 -> Mux/3

== system Smart_City_QCar2_VIRTUAL_car4/Rate Timing Plots/monitorTiming6 ==
  note: Timing Performance
  note: moniorTiming Module:
      |
      | This subsystem outputs the sample time and computation time of the model.
      |
      | Outputs:
      | sampleTime (s) n/a : Sample time (unfiltered and filtered) in seconds.
      | computationTime (s) n/a : Computation time (unfiltered and filtered) in seconds.
      |
      | Usage:
      | Compare the Sample Time (s) output to a constant (qc_get_step_size) to monitor whether or not the desired sample time is being achieved. The Computation Time (s) values should be lower than the corresponding sample time value to ensure that the solver has enough time per time step.
  Computation Time : quarc_library/Sources/Time/Computation Time  sample_time=NN_Sample_Time  use_model=on  use_cpu_time=off
  Constant : Constant  Value=NN_Sample_Time  SampleTime=-1
  Mux : Mux  Inputs=3
  Sample Time : quarc_library/Sources/Time/Sample Time  Priority=-99  sample_time=NN_Sample_Time
  Timing (s) : Outport  VectorParamsAs1DForOutWhenUnconnected=off
  wires:
  Computation Time/1 -> Mux/3
  Mux/1 -> Timing (s)/1
  Sample Time/1 -> Mux/1
  Constant/1 -> Mux/2
